simulink model "problema1"  (R2021a)
settings: Solver=VariableStepAuto  StartTime=0.0  StopTime=10.0  RelTol=1e-3
libraries: dspadpt3 x1
settings Model: Creator=Irek  LastModifiedBy=Irek

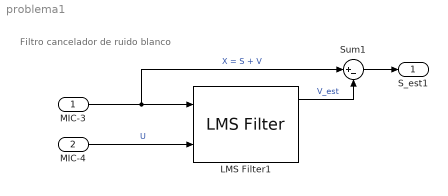
== system problema1 ==
  note: Filtro cancelador de ruido blanco
  MIC-3 : Inport
  MIC-4 : Inport  Port=2
  LMS Filter1 : dspadpt3/LMS Filter  Algo=LMS  L=32  stepflag=Dialog  mu=0.1  leakage=1.0  ic=0  Adapt=off  resetflag=None  weights=on  addnparflag=off  roundingMode=Floor  overflowMode=off  secondCoeffMode=Binary point scaling  secondCoeffWordLength=2  secondCoeffFracLength=15  prodOutput2Mode=Binary point scaling  prodOutput2FracLength=20  prodOutput3Mode=Binary point scaling  prodOutput3FracLength=20  prodOutput4Mode=Binary point scaling  prodOutput4FracLength=20  quotientMode=Binary point scaling  quotientFracLength=20  accum2Mode=Binary point scaling  accum2FracLength=20
      settings: SourceProductBaseCode=DS
  Sum1 : Sum  Inputs=|+-
  S_est1 : Outport
  wires:
  Sum1/1 -> S_est1/1
  LMS Filter1/1 -> Sum1/2  "V_est"
  MIC-4/1 -> LMS Filter1/2  "U"
  MIC-3/1 -> Sum1/1, LMS Filter1/1  "X = S + V"
